simulink library "ssc_Probes_2016a_org"  (Simulink 10.0)
settings: Solver=ode45  StartTime=0.0  StopTime=10.0  RelTol=1e-3  EnableMultiTasking=on
libraries: fl_lib x64, nesl_utility x64, pe_lib x9
(part 3 of 3)

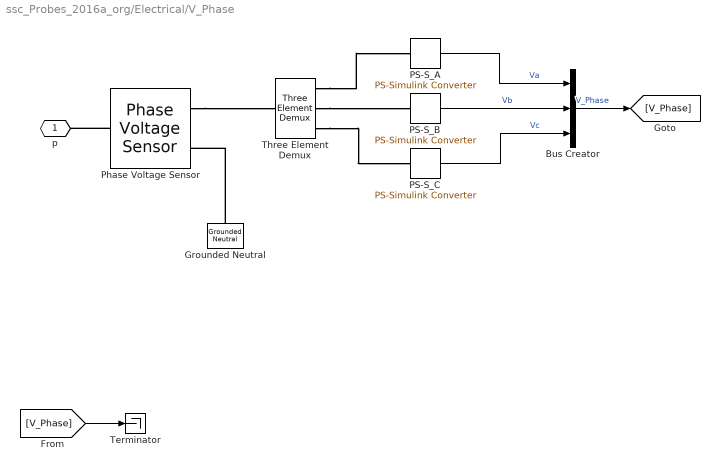
== system ssc_Probes_2016a_org/Electrical/V_Phase ==
  Bus Creator : BusCreator  Inputs=3
  Grounded Neutral : pe_lib/Connections/Grounded Neutral
      settings: SourceProductName=Simscape Electrical  SourceProductBaseCode=PS
  PS-S_A : nesl_utility/PS-Simulink Converter  PhysicalDomain=network_engine_domain  SubClassName=ps_output  LeftPortType=input  RightPortType=output  PseudoPeriodic=off  Frequencies=[]  Unit=V  AffineConversion=off
  PS-S_B : nesl_utility/PS-Simulink Converter  PhysicalDomain=network_engine_domain  SubClassName=ps_output  LeftPortType=input  RightPortType=output  PseudoPeriodic=off  Frequencies=[]  Unit=V  AffineConversion=off
  PS-S_C : nesl_utility/PS-Simulink Converter  PhysicalDomain=network_engine_domain  SubClassName=ps_output  LeftPortType=input  RightPortType=output  PseudoPeriodic=off  Frequencies=[]  Unit=V  AffineConversion=off
  Phase Voltage Sensor : pe_lib/Sensors/Phase Voltage Sensor
      settings: SourceProductName=Simscape Electrical  SourceProductBaseCode=PS
  Terminator : Terminator
  Three Element Demux : pe_lib/Sensors/Three Element Demux
      settings: SourceProductName=Simscape Electrical  SourceProductBaseCode=PS
  p : PMIOPort  Side=Left
  wires:
  [V_Phase] -> Terminator/1
  PS-S_A/1 -> Bus Creator/1  "Va"
  PS-S_B/1 -> Bus Creator/2  "Vb"
  PS-S_C/1 -> Bus Creator/3  "Vc"
  Bus Creator/1 -> [V_Phase]  "V_Phase"
  connections:
  Phase Voltage Sensor/LConn1 -- p/RConn1
  Three Element Demux/RConn3 -- PS-S_C/LConn1
  Three Element Demux/RConn1 -- PS-S_A/LConn1
  Three Element Demux/RConn2 -- PS-S_B/LConn1
  Phase Voltage Sensor/RConn1 -- Three Element Demux/LConn1
  Grounded Neutral/LConn1 -- Phase Voltage Sensor/RConn2

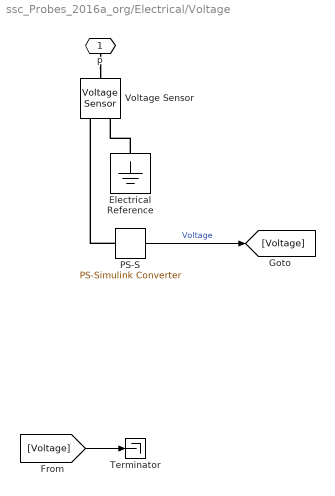
== system ssc_Probes_2016a_org/Electrical/Voltage ==
  Electrical Reference : fl_lib/Electrical/Electrical Elements/Electrical Reference
  PS-S : nesl_utility/PS-Simulink Converter  PhysicalDomain=network_engine_domain  SubClassName=ps_output  LeftPortType=input  RightPortType=output  PseudoPeriodic=off  Frequencies=[]  Unit=V  AffineConversion=off
  Terminator : Terminator
  Voltage Sensor : fl_lib/Electrical/Electrical Sensors/Voltage Sensor
  p : PMIOPort  Side=Left
  wires:
  PS-S/1 -> [Voltage]  "Voltage"
  [Voltage] -> Terminator/1
  connections:
  Electrical Reference/LConn1 -- Voltage Sensor/RConn2
  PS-S/LConn1 -- Voltage Sensor/RConn1
  p/RConn1 -- Voltage Sensor/LConn1

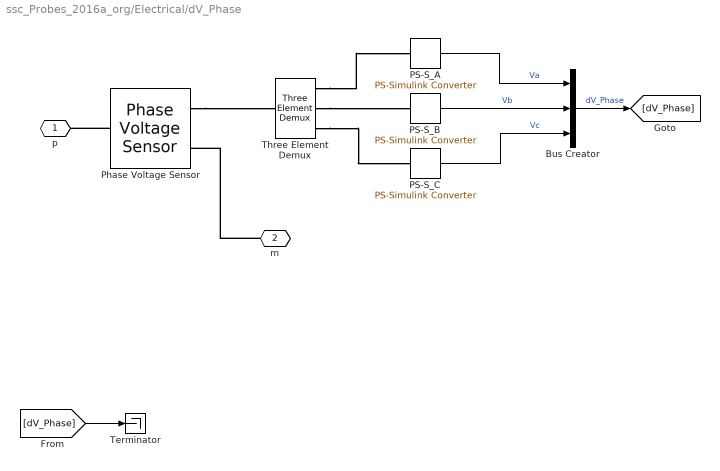
== system ssc_Probes_2016a_org/Electrical/dV_Phase ==
  Bus Creator : BusCreator  Inputs=3
  PS-S_A : nesl_utility/PS-Simulink Converter  PhysicalDomain=network_engine_domain  SubClassName=ps_output  LeftPortType=input  RightPortType=output  PseudoPeriodic=off  Frequencies=[]  Unit=V  AffineConversion=off
  PS-S_B : nesl_utility/PS-Simulink Converter  PhysicalDomain=network_engine_domain  SubClassName=ps_output  LeftPortType=input  RightPortType=output  PseudoPeriodic=off  Frequencies=[]  Unit=V  AffineConversion=off
  PS-S_C : nesl_utility/PS-Simulink Converter  PhysicalDomain=network_engine_domain  SubClassName=ps_output  LeftPortType=input  RightPortType=output  PseudoPeriodic=off  Frequencies=[]  Unit=V  AffineConversion=off
  Phase Voltage Sensor : pe_lib/Sensors/Phase Voltage Sensor
      settings: SourceProductName=Simscape Electrical  SourceProductBaseCode=PS
  Terminator : Terminator
  Three Element Demux : pe_lib/Sensors/Three Element Demux
      settings: SourceProductName=Simscape Electrical  SourceProductBaseCode=PS
  p : PMIOPort  Side=Left
  m : PMIOPort  Port=2  Side=Right
  wires:
  Bus Creator/1 -> [dV_Phase]  "dV_Phase"
  PS-S_C/1 -> Bus Creator/3  "Vc"
  PS-S_B/1 -> Bus Creator/2  "Vb"
  PS-S_A/1 -> Bus Creator/1  "Va"
  [dV_Phase] -> Terminator/1
  connections:
  m/RConn1 -- Phase Voltage Sensor/RConn2
  Phase Voltage Sensor/RConn1 -- Three Element Demux/LConn1
  Three Element Demux/RConn2 -- PS-S_B/LConn1
  Three Element Demux/RConn1 -- PS-S_A/LConn1
  Three Element Demux/RConn3 -- PS-S_C/LConn1
  Phase Voltage Sensor/LConn1 -- p/RConn1

== system ssc_Probes_2016a_org/Electrical/dVoltage ==
  PS-S : nesl_utility/PS-Simulink Converter  PhysicalDomain=network_engine_domain  SubClassName=ps_output  LeftPortType=input  RightPortType=output  PseudoPeriodic=off  Frequencies=[]  Unit=V  AffineConversion=off
  Terminator : Terminator
  Voltage Sensor : fl_lib/Electrical/Electrical Sensors/Voltage Sensor
  p : PMIOPort  Side=Left
  m : PMIOPort  Port=2  Side=Right
  wires:
  PS-S/1 -> [dVoltage]  "dVoltage"
  [dVoltage] -> Terminator/1
  connections:
  p/RConn1 -- Voltage Sensor/LConn1
  PS-S/LConn1 -- Voltage Sensor/RConn1
  m/RConn1 -- Voltage Sensor/RConn2

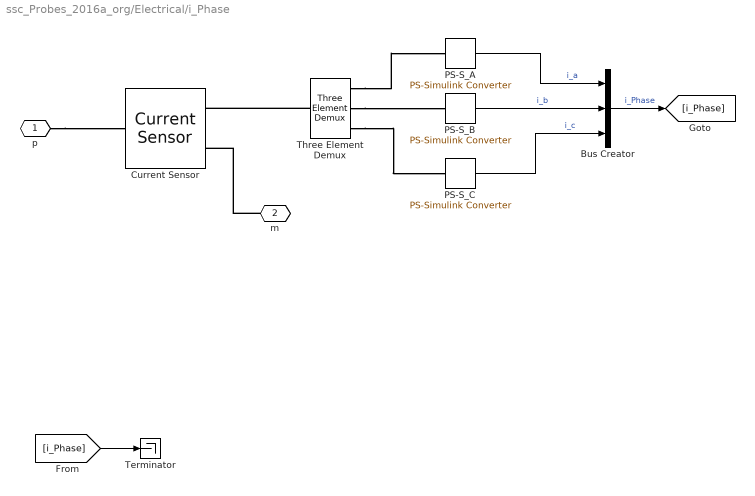
== system ssc_Probes_2016a_org/Electrical/i_Phase ==
  Bus Creator : BusCreator  Inputs=3
  Current Sensor : pe_lib/Sensors/Current Sensor
      settings: SourceProductName=Simscape Electrical  SourceProductBaseCode=PS
  PS-S_A : nesl_utility/PS-Simulink Converter  PhysicalDomain=network_engine_domain  SubClassName=ps_output  LeftPortType=input  RightPortType=output  PseudoPeriodic=off  Frequencies=[]  Unit=A  AffineConversion=off
  PS-S_B : nesl_utility/PS-Simulink Converter  PhysicalDomain=network_engine_domain  SubClassName=ps_output  LeftPortType=input  RightPortType=output  PseudoPeriodic=off  Frequencies=[]  Unit=A  AffineConversion=off
  PS-S_C : nesl_utility/PS-Simulink Converter  PhysicalDomain=network_engine_domain  SubClassName=ps_output  LeftPortType=input  RightPortType=output  PseudoPeriodic=off  Frequencies=[]  Unit=A  AffineConversion=off
  Terminator : Terminator
  Three Element Demux : pe_lib/Sensors/Three Element Demux
      settings: SourceProductName=Simscape Electrical  SourceProductBaseCode=PS
  p : PMIOPort  Side=Left
  m : PMIOPort  Port=2  Side=Right
  wires:
  [i_Phase] -> Terminator/1
  PS-S_A/1 -> Bus Creator/1  "i_a"
  PS-S_B/1 -> Bus Creator/2  "i_b"
  PS-S_C/1 -> Bus Creator/3  "i_c"
  Bus Creator/1 -> [i_Phase]  "i_Phase"
  connections:
  m/RConn1 -- Current Sensor/RConn2
  p/RConn1 -- Current Sensor/LConn1
  Three Element Demux/RConn3 -- PS-S_C/LConn1
  Three Element Demux/RConn2 -- PS-S_B/LConn1
  Three Element Demux/RConn1 -- PS-S_A/LConn1
  Three Element Demux/LConn1 -- Current Sensor/RConn1

== system ssc_Probes_2016a_org/Hydraulic/Flow ==
  Ideal Hydraulic Flow Rate Sensor : fl_lib/Hydraulic/Hydraulic Sensors/Hydraulic Flow Rate Sensor
      settings: SourceProductName=Simscape
  PS-S : nesl_utility/PS-Simulink Converter  PhysicalDomain=network_engine_domain  SubClassName=ps_output  LeftPortType=input  RightPortType=output  PseudoPeriodic=off  Frequencies=[]  Unit=m^3/s  AffineConversion=off
  Terminator : Terminator
  A : PMIOPort  Side=Left
  B : PMIOPort  Port=2  Side=Right
  wires:
  PS-S/1 -> [Flow]  "Flow"
  [Flow] -> Terminator/1
  connections:
  B/RConn1 -- Ideal Hydraulic Flow Rate Sensor/RConn2
  Ideal Hydraulic Flow Rate Sensor/RConn1 -- PS-S/LConn1
  A/RConn1 -- Ideal Hydraulic Flow Rate Sensor/LConn1

== system ssc_Probes_2016a_org/Hydraulic/Pressure ==
  Hydraulic Reference : fl_lib/Hydraulic/Hydraulic Elements/Hydraulic Reference
      settings: SourceProductName=Simscape
  Ideal Hydraulic Pressure Sensor : fl_lib/Hydraulic/Hydraulic Sensors/Hydraulic Pressure Sensor
      settings: SourceProductName=Simscape
  PS-S : nesl_utility/PS-Simulink Converter  PhysicalDomain=network_engine_domain  SubClassName=ps_output  LeftPortType=input  RightPortType=output  PseudoPeriodic=off  Frequencies=[]  Unit=Pa  AffineConversion=off
  Terminator : Terminator
  A : PMIOPort  Side=Left
  wires:
  PS-S/1 -> [Pressure]  "Pressure"
  [Pressure] -> Terminator/1
  connections:
  PS-S/LConn1 -- Ideal Hydraulic Pressure Sensor/RConn2
  Hydraulic Reference/LConn1 -- Ideal Hydraulic Pressure Sensor/RConn1
  A/RConn1 -- Ideal Hydraulic Pressure Sensor/LConn1

== system ssc_Probes_2016a_org/Hydraulic/dPressure ==
  Ideal Hydraulic Pressure Sensor : fl_lib/Hydraulic/Hydraulic Sensors/Hydraulic Pressure Sensor
      settings: SourceProductName=Simscape
  PS-S : nesl_utility/PS-Simulink Converter  PhysicalDomain=network_engine_domain  SubClassName=ps_output  LeftPortType=input  RightPortType=output  PseudoPeriodic=off  Frequencies=[]  Unit=Pa  AffineConversion=off
  Terminator : Terminator
  A : PMIOPort  Side=Left
  B : PMIOPort  Port=2  Side=Right
  wires:
  PS-S/1 -> [dPressure]  "dPressure"
  [dPressure] -> Terminator/1
  connections:
  A/RConn1 -- Ideal Hydraulic Pressure Sensor/LConn1
  B/RConn1 -- Ideal Hydraulic Pressure Sensor/RConn1
  PS-S/LConn1 -- Ideal Hydraulic Pressure Sensor/RConn2

== system ssc_Probes_2016a_org/Magnetic/Flux ==
  Flux Sensor : fl_lib/Magnetic/Magnetic Sensors/Flux Sensor
      settings: SourceProductName=Simscape  SourceProductBaseCode=SS
  PS-S : nesl_utility/PS-Simulink Converter  PhysicalDomain=network_engine_domain  SubClassName=ps_output  LeftPortType=input  RightPortType=output  PseudoPeriodic=off  Frequencies=[]  Unit=Wb  AffineConversion=off
  Terminator : Terminator
  N : PMIOPort  Side=Left
  S : PMIOPort  Port=2  Side=Right
  wires:
  PS-S/1 -> [Flux]  "Flux"
  [Flux] -> Terminator/1
  connections:
  N/RConn1 -- Flux Sensor/LConn1
  Flux Sensor/RConn1 -- PS-S/LConn1
  S/RConn1 -- Flux Sensor/RConn2

== system ssc_Probes_2016a_org/Magnetic/MMF ==
  MMF Sensor : fl_lib/Magnetic/Magnetic Sensors/MMF Sensor
      settings: SourceProductName=Simscape  SourceProductBaseCode=SS
  Magnetic Reference : fl_lib/Magnetic/Magnetic Elements/Magnetic Reference
      settings: SourceProductName=Simscape  SourceProductBaseCode=SS
  PS-S : nesl_utility/PS-Simulink Converter  PhysicalDomain=network_engine_domain  SubClassName=ps_output  LeftPortType=input  RightPortType=output  PseudoPeriodic=off  Frequencies=[]  Unit=A  AffineConversion=off
  Terminator : Terminator
  N : PMIOPort  Side=Left
  wires:
  PS-S/1 -> [MMF]  "MMF"
  [MMF] -> Terminator/1
  connections:
  Magnetic Reference/LConn1 -- MMF Sensor/RConn2
  MMF Sensor/RConn1 -- PS-S/LConn1
  N/RConn1 -- MMF Sensor/LConn1

== system ssc_Probes_2016a_org/Magnetic/dMMF ==
  MMF Sensor : fl_lib/Magnetic/Magnetic Sensors/MMF Sensor
      settings: SourceProductName=Simscape  SourceProductBaseCode=SS
  PS-S : nesl_utility/PS-Simulink Converter  PhysicalDomain=network_engine_domain  SubClassName=ps_output  LeftPortType=input  RightPortType=output  PseudoPeriodic=off  Frequencies=[]  Unit=A  AffineConversion=off
  Terminator : Terminator
  N : PMIOPort  Side=Left
  S : PMIOPort  Port=2  Side=Right
  wires:
  PS-S/1 -> [dMMF]  "dMMF"
  [dMMF] -> Terminator/1
  connections:
  N/RConn1 -- MMF Sensor/LConn1
  MMF Sensor/RConn1 -- PS-S/LConn1
  S/RConn1 -- MMF Sensor/RConn2

== system ssc_Probes_2016a_org/Mechanical/AngVel ==
  Ideal Rotational Motion Sensor : fl_lib/Mechanical/Mechanical Sensors/Ideal Rotational Motion Sensor  offset=0 rad
  Mechanical Rotational Reference : fl_lib/Mechanical/Rotational Elements/Mechanical Rotational Reference
  PS-S : nesl_utility/PS-Simulink Converter  PhysicalDomain=network_engine_domain  SubClassName=ps_output  LeftPortType=input  RightPortType=output  PseudoPeriodic=off  Frequencies=[]  Unit=rad/s  AffineConversion=off
  Terminator : Terminator
  R : PMIOPort  Side=Left
  wires:
  PS-S/1 -> [AngVel]  "AngVel"
  [AngVel] -> Terminator/1
  connections:
  Ideal Rotational Motion Sensor/RConn2 -- PS-S/LConn1
  Mechanical Rotational Reference/LConn1 -- Ideal Rotational Motion Sensor/RConn1
  R/RConn1 -- Ideal Rotational Motion Sensor/LConn1

== system ssc_Probes_2016a_org/Mechanical/Angle ==
  Ideal Rotational Motion Sensor : fl_lib/Mechanical/Mechanical Sensors/Ideal Rotational Motion Sensor  offset=0 rad
  Mechanical Rotational Reference : fl_lib/Mechanical/Rotational Elements/Mechanical Rotational Reference
  PS-S : nesl_utility/PS-Simulink Converter  PhysicalDomain=network_engine_domain  SubClassName=ps_output  LeftPortType=input  RightPortType=output  PseudoPeriodic=off  Frequencies=[]  Unit=rad  AffineConversion=off
  Terminator : Terminator
  R : PMIOPort  Side=Left
  wires:
  PS-S/1 -> [Angle]  "Angle"
  [Angle] -> Terminator/1
  connections:
  R/RConn1 -- Ideal Rotational Motion Sensor/LConn1
  Mechanical Rotational Reference/LConn1 -- Ideal Rotational Motion Sensor/RConn1
  PS-S/LConn1 -- Ideal Rotational Motion Sensor/RConn3

== system ssc_Probes_2016a_org/Mechanical/Force ==
  Ideal Force Sensor : fl_lib/Mechanical/Mechanical Sensors/Ideal Force Sensor
  PS-S : nesl_utility/PS-Simulink Converter  PhysicalDomain=network_engine_domain  SubClassName=ps_output  LeftPortType=input  RightPortType=output  PseudoPeriodic=off  Frequencies=[]  Unit=N  AffineConversion=off
  Terminator : Terminator
  R : PMIOPort  Side=Left
  C : PMIOPort  Port=2  Side=Right
  wires:
  PS-S/1 -> [Force]  "Force"
  [Force] -> Terminator/1
  connections:
  C/RConn1 -- Ideal Force Sensor/RConn1
  Ideal Force Sensor/RConn2 -- PS-S/LConn1
  R/RConn1 -- Ideal Force Sensor/LConn1

== system ssc_Probes_2016a_org/Mechanical/Position ==
  Ideal Translational Motion Sensor : fl_lib/Mechanical/Mechanical Sensors/Ideal Translational Motion Sensor  offset=0 m
  Mechanical Translational Reference : fl_lib/Mechanical/Translational Elements/Mechanical Translational Reference
  PS-S : nesl_utility/PS-Simulink Converter  PhysicalDomain=network_engine_domain  SubClassName=ps_output  LeftPortType=input  RightPortType=output  PseudoPeriodic=off  Frequencies=[]  Unit=m  AffineConversion=off
  Terminator : Terminator
  R : PMIOPort  Side=Left
  wires:
  PS-S/1 -> [Position]  "Position"
  [Position] -> Terminator/1
  connections:
  PS-S/LConn1 -- Ideal Translational Motion Sensor/RConn3
  Mechanical Translational Reference/LConn1 -- Ideal Translational Motion Sensor/RConn1
  R/RConn1 -- Ideal Translational Motion Sensor/LConn1

== system ssc_Probes_2016a_org/Mechanical/Torque ==
  Ideal Torque Sensor : fl_lib/Mechanical/Mechanical Sensors/Ideal Torque Sensor
  PS-S : nesl_utility/PS-Simulink Converter  PhysicalDomain=network_engine_domain  SubClassName=ps_output  LeftPortType=input  RightPortType=output  PseudoPeriodic=off  Frequencies=[]  Unit=N*m  AffineConversion=off
  Terminator : Terminator
  R : PMIOPort  Side=Left
  C : PMIOPort  Port=2  Side=Right
  wires:
  PS-S/1 -> [Torque]  "Torque"
  [Torque] -> Terminator/1
  connections:
  R/RConn1 -- Ideal Torque Sensor/LConn1
  Ideal Torque Sensor/RConn2 -- PS-S/LConn1
  C/RConn1 -- Ideal Torque Sensor/RConn1

== system ssc_Probes_2016a_org/Mechanical/Velocity ==
  Ideal Translational Motion Sensor : fl_lib/Mechanical/Mechanical Sensors/Ideal Translational Motion Sensor  offset=0 m
  Mechanical Translational Reference : fl_lib/Mechanical/Translational Elements/Mechanical Translational Reference
  PS-S : nesl_utility/PS-Simulink Converter  PhysicalDomain=network_engine_domain  SubClassName=ps_output  LeftPortType=input  RightPortType=output  PseudoPeriodic=off  Frequencies=[]  Unit=m/s  AffineConversion=off
  Terminator : Terminator
  R : PMIOPort  Side=Left
  wires:
  PS-S/1 -> [Velocity]  "Velocity"
  [Velocity] -> Terminator/1
  connections:
  Ideal Translational Motion Sensor/RConn2 -- PS-S/LConn1
  R/RConn1 -- Ideal Translational Motion Sensor/LConn1
  Mechanical Translational Reference/LConn1 -- Ideal Translational Motion Sensor/RConn1

== system ssc_Probes_2016a_org/Mechanical/dAngVel ==
  Ideal Rotational Motion Sensor : fl_lib/Mechanical/Mechanical Sensors/Ideal Rotational Motion Sensor  offset=0 rad
  PS-S : nesl_utility/PS-Simulink Converter  PhysicalDomain=network_engine_domain  SubClassName=ps_output  LeftPortType=input  RightPortType=output  PseudoPeriodic=off  Frequencies=[]  Unit=rad/s  AffineConversion=off
  Terminator : Terminator
  R : PMIOPort  Side=Left
  C : PMIOPort  Port=2  Side=Right
  wires:
  PS-S/1 -> [dAngVel]  "dAngVel"
  [dAngVel] -> Terminator/1
  connections:
  R/RConn1 -- Ideal Rotational Motion Sensor/LConn1
  C/RConn1 -- Ideal Rotational Motion Sensor/RConn1
  Ideal Rotational Motion Sensor/RConn2 -- PS-S/LConn1

== system ssc_Probes_2016a_org/Mechanical/dAngle ==
  Ideal Rotational Motion Sensor : fl_lib/Mechanical/Mechanical Sensors/Ideal Rotational Motion Sensor  offset=0 rad
  PS-S : nesl_utility/PS-Simulink Converter  PhysicalDomain=network_engine_domain  SubClassName=ps_output  LeftPortType=input  RightPortType=output  PseudoPeriodic=off  Frequencies=[]  Unit=rad  AffineConversion=off
  Terminator : Terminator
  R : PMIOPort  Side=Left
  C : PMIOPort  Port=2  Side=Right
  wires:
  PS-S/1 -> [dAngle]  "dAngle"
  [dAngle] -> Terminator/1
  connections:
  PS-S/LConn1 -- Ideal Rotational Motion Sensor/RConn3
  C/RConn1 -- Ideal Rotational Motion Sensor/RConn1
  R/RConn1 -- Ideal Rotational Motion Sensor/LConn1

== system ssc_Probes_2016a_org/Mechanical/dPosition ==
  Ideal Translational Motion Sensor : fl_lib/Mechanical/Mechanical Sensors/Ideal Translational Motion Sensor  offset=0 m
  PS-S : nesl_utility/PS-Simulink Converter  PhysicalDomain=network_engine_domain  SubClassName=ps_output  LeftPortType=input  RightPortType=output  PseudoPeriodic=off  Frequencies=[]  Unit=m  AffineConversion=off
  Terminator : Terminator
  R : PMIOPort  Side=Left
  C : PMIOPort  Port=2  Side=Right
  wires:
  PS-S/1 -> [dPosition]  "dPosition"
  [dPosition] -> Terminator/1
  connections:
  R/RConn1 -- Ideal Translational Motion Sensor/LConn1
  C/RConn1 -- Ideal Translational Motion Sensor/RConn1
  PS-S/LConn1 -- Ideal Translational Motion Sensor/RConn3

== system ssc_Probes_2016a_org/Mechanical/dVelocity ==
  Ideal Translational Motion Sensor : fl_lib/Mechanical/Mechanical Sensors/Ideal Translational Motion Sensor  offset=0 m
  PS-S : nesl_utility/PS-Simulink Converter  PhysicalDomain=network_engine_domain  SubClassName=ps_output  LeftPortType=input  RightPortType=output  PseudoPeriodic=off  Frequencies=[]  Unit=m/s  AffineConversion=off
  Terminator : Terminator
  R : PMIOPort  Side=Left
  C : PMIOPort  Port=2  Side=Right
  wires:
  PS-S/1 -> [dVelocity]  "dVelocity"
  [dVelocity] -> Terminator/1
  connections:
  C/RConn1 -- Ideal Translational Motion Sensor/RConn1
  R/RConn1 -- Ideal Translational Motion Sensor/LConn1
  PS-S/LConn1 -- Ideal Translational Motion Sensor/RConn2

== system ssc_Probes_2016a_org/Pneumatic/AbsPressure ==
  PS-S : nesl_utility/PS-Simulink Converter  PhysicalDomain=network_engine_domain  SubClassName=ps_output  LeftPortType=input  RightPortType=output  PseudoPeriodic=off  Frequencies=[]  Unit=Pa  AffineConversion=off
  Pneumatic Absolute Reference : fl_lib/Pneumatic/Pneumatic Elements/Pneumatic Absolute Reference
      settings: SourceProductName=Simscape  SourceProductBaseCode=SS
  Pneumatic Pressure & Temperature Sensor : fl_lib/Pneumatic/Pneumatic Sensors/Pneumatic Pressure & Temperature Sensor
      settings: SourceProductName=Simscape  SourceProductBaseCode=SS
  Terminator : Terminator
  A : PMIOPort  Side=Left
  wires:
  PS-S/1 -> [AbsPressure]  "AbsPressure"
  [AbsPressure] -> Terminator/1
  connections:
  A/RConn1 -- Pneumatic Pressure & Temperature Sensor/LConn1
  Pneumatic Absolute Reference/LConn1 -- Pneumatic Pressure & Temperature Sensor/RConn1
  PS-S/LConn1 -- Pneumatic Pressure & Temperature Sensor/RConn2

== system ssc_Probes_2016a_org/Pneumatic/AbsTemperature ==
  PS-S : nesl_utility/PS-Simulink Converter  PhysicalDomain=network_engine_domain  SubClassName=ps_output  LeftPortType=input  RightPortType=output  PseudoPeriodic=off  Frequencies=[]  Unit=K  AffineConversion=off
  Pneumatic Absolute Reference : fl_lib/Pneumatic/Pneumatic Elements/Pneumatic Absolute Reference
      settings: SourceProductName=Simscape  SourceProductBaseCode=SS
  Pneumatic Pressure & Temperature Sensor : fl_lib/Pneumatic/Pneumatic Sensors/Pneumatic Pressure & Temperature Sensor
      settings: SourceProductName=Simscape  SourceProductBaseCode=SS
  Terminator : Terminator
  A : PMIOPort  Side=Left
  wires:
  PS-S/1 -> [AbsTemperature]  "AbsTemperature"
  [AbsTemperature] -> Terminator/1
  connections:
  PS-S/LConn1 -- Pneumatic Pressure & Temperature Sensor/RConn3
  Pneumatic Absolute Reference/LConn1 -- Pneumatic Pressure & Temperature Sensor/RConn1
  A/RConn1 -- Pneumatic Pressure & Temperature Sensor/LConn1

== system ssc_Probes_2016a_org/Pneumatic/AtmTemperature ==
  PS-S : nesl_utility/PS-Simulink Converter  PhysicalDomain=network_engine_domain  SubClassName=ps_output  LeftPortType=input  RightPortType=output  PseudoPeriodic=off  Frequencies=[]  Unit=K  AffineConversion=off
  Pneumatic Atmospheric Reference : fl_lib/Pneumatic/Pneumatic Elements/Pneumatic Atmospheric Reference
      settings: SourceProductName=Simscape  SourceProductBaseCode=SS
  Pneumatic Pressure & Temperature Sensor : fl_lib/Pneumatic/Pneumatic Sensors/Pneumatic Pressure & Temperature Sensor
      settings: SourceProductName=Simscape  SourceProductBaseCode=SS
  Terminator : Terminator
  A : PMIOPort  Side=Left
  wires:
  PS-S/1 -> [AtmTemperature]  "AtmTemperature"
  [AtmTemperature] -> Terminator/1
  connections:
  A/RConn1 -- Pneumatic Pressure & Temperature Sensor/LConn1
  Pneumatic Atmospheric Reference/LConn1 -- Pneumatic Pressure & Temperature Sensor/RConn1
  PS-S/LConn1 -- Pneumatic Pressure & Temperature Sensor/RConn3

== system ssc_Probes_2016a_org/Pneumatic/GasHeatFlow ==
  PS-S : nesl_utility/PS-Simulink Converter  PhysicalDomain=network_engine_domain  SubClassName=ps_output  LeftPortType=input  RightPortType=output  PseudoPeriodic=off  Frequencies=[]  Unit=J/s  AffineConversion=off
  Pneumatic Mass & Heat Flow Sensor : fl_lib/Pneumatic/Pneumatic Sensors/Pneumatic Mass & Heat Flow Sensor
      settings: SourceProductName=Simscape  SourceProductBaseCode=SS
  Terminator : Terminator
  A : PMIOPort  Side=Left
  B : PMIOPort  Port=2  Side=Right
  wires:
  PS-S/1 -> [GasHeatFlow]  "GasHeatFlow"
  [GasHeatFlow] -> Terminator/1
  connections:
  PS-S/LConn1 -- Pneumatic Mass & Heat Flow Sensor/RConn3
  B/RConn1 -- Pneumatic Mass & Heat Flow Sensor/RConn1
  A/RConn1 -- Pneumatic Mass & Heat Flow Sensor/LConn1

== system ssc_Probes_2016a_org/Pneumatic/GaugePressure ==
  PS-S : nesl_utility/PS-Simulink Converter  PhysicalDomain=network_engine_domain  SubClassName=ps_output  LeftPortType=input  RightPortType=output  PseudoPeriodic=off  Frequencies=[]  Unit=Pa  AffineConversion=off
  Pneumatic Atmospheric Reference : fl_lib/Pneumatic/Pneumatic Elements/Pneumatic Atmospheric Reference
      settings: SourceProductName=Simscape  SourceProductBaseCode=SS
  Pneumatic Pressure & Temperature Sensor : fl_lib/Pneumatic/Pneumatic Sensors/Pneumatic Pressure & Temperature Sensor
      settings: SourceProductName=Simscape  SourceProductBaseCode=SS
  Terminator : Terminator
  A : PMIOPort  Side=Left
  wires:
  PS-S/1 -> [GaugePressure]  "GaugePressure"
  [GaugePressure] -> Terminator/1
  connections:
  PS-S/LConn1 -- Pneumatic Pressure & Temperature Sensor/RConn2
  Pneumatic Atmospheric Reference/LConn1 -- Pneumatic Pressure & Temperature Sensor/RConn1
  A/RConn1 -- Pneumatic Pressure & Temperature Sensor/LConn1

== system ssc_Probes_2016a_org/Pneumatic/MassFlow ==
  PS-S : nesl_utility/PS-Simulink Converter  PhysicalDomain=network_engine_domain  SubClassName=ps_output  LeftPortType=input  RightPortType=output  PseudoPeriodic=off  Frequencies=[]  Unit=kg/s  AffineConversion=off
  Pneumatic Mass & Heat Flow Sensor : fl_lib/Pneumatic/Pneumatic Sensors/Pneumatic Mass & Heat Flow Sensor
      settings: SourceProductName=Simscape  SourceProductBaseCode=SS
  Terminator : Terminator
  A : PMIOPort  Side=Left
  B : PMIOPort  Port=2  Side=Right
  wires:
  PS-S/1 -> [MassFlow]  "MassFlow"
  [MassFlow] -> Terminator/1
  connections:
  A/RConn1 -- Pneumatic Mass & Heat Flow Sensor/LConn1
  Pneumatic Mass & Heat Flow Sensor/RConn2 -- PS-S/LConn1
  B/RConn1 -- Pneumatic Mass & Heat Flow Sensor/RConn1

== system ssc_Probes_2016a_org/Pneumatic/dGasPressure ==
  PS-S : nesl_utility/PS-Simulink Converter  PhysicalDomain=network_engine_domain  SubClassName=ps_output  LeftPortType=input  RightPortType=output  PseudoPeriodic=off  Frequencies=[]  Unit=Pa  AffineConversion=off
  Pneumatic Pressure & Temperature Sensor : fl_lib/Pneumatic/Pneumatic Sensors/Pneumatic Pressure & Temperature Sensor
      settings: SourceProductName=Simscape  SourceProductBaseCode=SS
  Terminator : Terminator
  A : PMIOPort  Side=Left
  B : PMIOPort  Port=2  Side=Right
  wires:
  PS-S/1 -> [dGasPressure]  "dGasPressure"
  [dGasPressure] -> Terminator/1
  connections:
  A/RConn1 -- Pneumatic Pressure & Temperature Sensor/LConn1
  B/RConn1 -- Pneumatic Pressure & Temperature Sensor/RConn1
  Pneumatic Pressure & Temperature Sensor/RConn2 -- PS-S/LConn1

== system ssc_Probes_2016a_org/Pneumatic/dGasTemperature ==
  PS-S : nesl_utility/PS-Simulink Converter  PhysicalDomain=network_engine_domain  SubClassName=ps_output  LeftPortType=input  RightPortType=output  PseudoPeriodic=off  Frequencies=[]  Unit=K  AffineConversion=off
  Pneumatic Pressure & Temperature Sensor : fl_lib/Pneumatic/Pneumatic Sensors/Pneumatic Pressure & Temperature Sensor
      settings: SourceProductName=Simscape  SourceProductBaseCode=SS
  Terminator : Terminator
  A : PMIOPort  Side=Left
  B : PMIOPort  Port=2  Side=Right
  wires:
  PS-S/1 -> [dGasTemperature]  "dGasTemperature"
  [dGasTemperature] -> Terminator/1
  connections:
  PS-S/LConn1 -- Pneumatic Pressure & Temperature Sensor/RConn3
  B/RConn1 -- Pneumatic Pressure & Temperature Sensor/RConn1
  A/RConn1 -- Pneumatic Pressure & Temperature Sensor/LConn1

== system ssc_Probes_2016a_org/Thermal/HeatFlow ==
  Ideal Heat Flow Sensor : fl_lib/Thermal/Thermal Sensors/Ideal Heat Flow Sensor
      settings: SourceProductName=Simscape  SourceProductBaseCode=SS
  PS-S : nesl_utility/PS-Simulink Converter  PhysicalDomain=network_engine_domain  SubClassName=ps_output  LeftPortType=input  RightPortType=output  PseudoPeriodic=off  Frequencies=[]  Unit=J/s  AffineConversion=off
  Terminator : Terminator
  A : PMIOPort  Side=Left
  B : PMIOPort  Port=2  Side=Right
  wires:
  PS-S/1 -> [HeatFlow]  "HeatFlow"
  [HeatFlow] -> Terminator/1
  connections:
  A/RConn1 -- Ideal Heat Flow Sensor/LConn1
  Ideal Heat Flow Sensor/RConn1 -- PS-S/LConn1
  B/RConn1 -- Ideal Heat Flow Sensor/RConn2

== system ssc_Probes_2016a_org/Thermal/Temperature ==
  Ideal Temperature Sensor : fl_lib/Thermal/Thermal Sensors/Ideal Temperature Sensor
      settings: SourceProductName=Simscape  SourceProductBaseCode=SS
  PS-S : nesl_utility/PS-Simulink Converter  PhysicalDomain=network_engine_domain  SubClassName=ps_output  LeftPortType=input  RightPortType=output  PseudoPeriodic=off  Frequencies=[]  Unit=K  AffineConversion=off
  Terminator : Terminator
  Thermal Reference : fl_lib/Thermal/Thermal Elements/Thermal Reference
  A : PMIOPort  Side=Left
  wires:
  PS-S/1 -> [Temperature]  "Temperature"
  [Temperature] -> Terminator/1
  connections:
  A/RConn1 -- Ideal Temperature Sensor/LConn1
  Thermal Reference/LConn1 -- Ideal Temperature Sensor/RConn1
  PS-S/LConn1 -- Ideal Temperature Sensor/RConn2

== system ssc_Probes_2016a_org/Thermal/dTemperature ==
  Ideal Temperature Sensor : fl_lib/Thermal/Thermal Sensors/Ideal Temperature Sensor
      settings: SourceProductName=Simscape  SourceProductBaseCode=SS
  PS-S : nesl_utility/PS-Simulink Converter  PhysicalDomain=network_engine_domain  SubClassName=ps_output  LeftPortType=input  RightPortType=output  PseudoPeriodic=off  Frequencies=[]  Unit=K  AffineConversion=off
  Terminator : Terminator
  A : PMIOPort  Side=Left
  B : PMIOPort  Port=2  Side=Right
  wires:
  PS-S/1 -> [dTemperature]  "dTemperature"
  [dTemperature] -> Terminator/1
  connections:
  PS-S/LConn1 -- Ideal Temperature Sensor/RConn2
  B/RConn1 -- Ideal Temperature Sensor/RConn1
  A/RConn1 -- Ideal Temperature Sensor/LConn1

== system ssc_Probes_2016a_org/ThermalLiquid/AbsPressure_TL ==
  Absolute Reference (TL) : fl_lib/Thermal Liquid/Elements/Absolute Reference (TL)
      settings: SourceProductName=Simscape  SourceProductBaseCode=SS
  PS-S : nesl_utility/PS-Simulink Converter  PhysicalDomain=network_engine_domain  SubClassName=ps_output  LeftPortType=input  RightPortType=output  PseudoPeriodic=off  Frequencies=[]  Unit=Pa  AffineConversion=off
  Pressure & Temperature Sensor (TL) : fl_lib/Thermal Liquid/Sensors/Pressure & Temperature Sensor (TL)
      settings: SourceProductName=Simscape  SourceProductBaseCode=SS
  Terminator : Terminator
  A : PMIOPort  Side=Left
  wires:
  PS-S/1 -> [AbsPressure_TL]  "AbsPressure_TL"
  [AbsPressure_TL] -> Terminator/1
  connections:
  Absolute Reference (TL)/LConn1 -- Pressure & Temperature Sensor (TL)/RConn1
  Pressure & Temperature Sensor (TL)/LConn1 -- A/RConn1
  PS-S/LConn1 -- Pressure & Temperature Sensor (TL)/RConn2

== system ssc_Probes_2016a_org/ThermalLiquid/AbsTemperature_TL ==
  Absolute Reference (TL) : fl_lib/Thermal Liquid/Elements/Absolute Reference (TL)
      settings: SourceProductName=Simscape  SourceProductBaseCode=SS
  PS-S : nesl_utility/PS-Simulink Converter  PhysicalDomain=network_engine_domain  SubClassName=ps_output  LeftPortType=input  RightPortType=output  PseudoPeriodic=off  Frequencies=[]  Unit=K  AffineConversion=off
  Pressure & Temperature Sensor (TL) : fl_lib/Thermal Liquid/Sensors/Pressure & Temperature Sensor (TL)
      settings: SourceProductName=Simscape  SourceProductBaseCode=SS
  Terminator : Terminator
  A : PMIOPort  Side=Left
  wires:
  [AbsTemperature_TL] -> Terminator/1
  PS-S/1 -> [AbsTemperature_TL]  "AbsTemperature_TL"
  connections:
  PS-S/LConn1 -- Pressure & Temperature Sensor (TL)/RConn3
  Pressure & Temperature Sensor (TL)/LConn1 -- A/RConn1
  Absolute Reference (TL)/LConn1 -- Pressure & Temperature Sensor (TL)/RConn1

== system ssc_Probes_2016a_org/ThermalLiquid/MassFlow_TL ==
  Mass Flow Rate & Thermal Flux Sensor (TL) : fl_lib/Thermal Liquid/Sensors/Mass & Energy Flow Rate Sensor (TL)
      settings: SourceProductName=Simscape  SourceProductBaseCode=SS
  PS-S : nesl_utility/PS-Simulink Converter  PhysicalDomain=network_engine_domain  SubClassName=ps_output  LeftPortType=input  RightPortType=output  PseudoPeriodic=off  Frequencies=[]  Unit=kg/s  AffineConversion=off
  Terminator : Terminator
  A : PMIOPort  Side=Left
  B : PMIOPort  Port=2  Side=Right
  wires:
  [MassFlow_TL] -> Terminator/1
  PS-S/1 -> [MassFlow_TL]  "MassFlow_TL"
  connections:
  Mass Flow Rate & Thermal Flux Sensor (TL)/RConn1 -- B/RConn1
  PS-S/LConn1 -- Mass Flow Rate & Thermal Flux Sensor (TL)/RConn2
  Mass Flow Rate & Thermal Flux Sensor (TL)/LConn1 -- A/RConn1

== system ssc_Probes_2016a_org/ThermalLiquid/ThermalFlux_TL ==
  Mass Flow Rate & Thermal Flux Sensor (TL) : fl_lib/Thermal Liquid/Sensors/Mass & Energy Flow Rate Sensor (TL)
      settings: SourceProductName=Simscape  SourceProductBaseCode=SS
  PS-S : nesl_utility/PS-Simulink Converter  PhysicalDomain=network_engine_domain  SubClassName=ps_output  LeftPortType=input  RightPortType=output  PseudoPeriodic=off  Frequencies=[]  Unit=J/s  AffineConversion=off
  Terminator : Terminator
  A : PMIOPort  Side=Left
  B : PMIOPort  Port=2  Side=Right
  wires:
  PS-S/1 -> [ThermalFlux_TL]  "ThermalFlux_TL"
  [ThermalFlux_TL] -> Terminator/1
  connections:
  Mass Flow Rate & Thermal Flux Sensor (TL)/LConn1 -- A/RConn1
  Mass Flow Rate & Thermal Flux Sensor (TL)/RConn1 -- B/RConn1
  Mass Flow Rate & Thermal Flux Sensor (TL)/RConn3 -- PS-S/LConn1

== system ssc_Probes_2016a_org/ThermalLiquid/dPressure_TL ==
  PS-S : nesl_utility/PS-Simulink Converter  PhysicalDomain=network_engine_domain  SubClassName=ps_output  LeftPortType=input  RightPortType=output  PseudoPeriodic=off  Frequencies=[]  Unit=Pa  AffineConversion=off
  Pressure & Temperature Sensor (TL) : fl_lib/Thermal Liquid/Sensors/Pressure & Temperature Sensor (TL)
      settings: SourceProductName=Simscape  SourceProductBaseCode=SS
  Terminator : Terminator
  A : PMIOPort  Side=Left
  B : PMIOPort  Port=2  Side=Right
  wires:
  PS-S/1 -> [dPressure_TL]  "dPressure_TL"
  [dPressure_TL] -> Terminator/1
  connections:
  B/RConn1 -- Pressure & Temperature Sensor (TL)/RConn1
  Pressure & Temperature Sensor (TL)/LConn1 -- A/RConn1
  Pressure & Temperature Sensor (TL)/RConn2 -- PS-S/LConn1

== system ssc_Probes_2016a_org/ThermalLiquid/dTemperature_TL ==
  PS-S : nesl_utility/PS-Simulink Converter  PhysicalDomain=network_engine_domain  SubClassName=ps_output  LeftPortType=input  RightPortType=output  PseudoPeriodic=off  Frequencies=[]  Unit=K  AffineConversion=off
  Pressure & Temperature Sensor (TL) : fl_lib/Thermal Liquid/Sensors/Pressure & Temperature Sensor (TL)
      settings: SourceProductName=Simscape  SourceProductBaseCode=SS
  Terminator : Terminator
  A : PMIOPort  Side=Left
  B : PMIOPort  Port=2  Side=Right
  wires:
  [dTemperature_TL] -> Terminator/1
  PS-S/1 -> [dTemperature_TL]  "dTemperature_TL"
  connections:
  Pressure & Temperature Sensor (TL)/LConn1 -- A/RConn1
  B/RConn1 -- Pressure & Temperature Sensor (TL)/RConn1
  PS-S/LConn1 -- Pressure & Temperature Sensor (TL)/RConn3

== system ssc_Probes_2016a_org/TwoPhaseFluid/AbsPressure_2P ==
  Absolute Reference (2P) : fl_lib/Two-Phase Fluid/Elements/Absolute Reference (2P)
      settings: SourceProductName=Simscape  SourceProductBaseCode=SS
  PS-S : nesl_utility/PS-Simulink Converter  PhysicalDomain=network_engine_domain  SubClassName=ps_output  LeftPortType=input  RightPortType=output  PseudoPeriodic=off  Frequencies=[]  Unit=Pa  AffineConversion=off
  Pressure & Internal Energy Sensor (2P) : fl_lib/Two-Phase Fluid/Sensors/Pressure & Internal Energy Sensor (2P)
      settings: SourceProductName=Simscape  SourceProductBaseCode=SS
  Terminator : Terminator
  A : PMIOPort  Side=Left
  wires:
  PS-S/1 -> [AbsPressure_2P]  "AbsPressure_2P"
  [AbsPressure_2P] -> Terminator/1
  connections:
  Pressure & Internal Energy Sensor (2P)/LConn1 -- A/RConn1
  Pressure & Internal Energy Sensor (2P)/RConn2 -- PS-S/LConn1
  Absolute Reference (2P)/LConn1 -- Pressure & Internal Energy Sensor (2P)/RConn1

== system ssc_Probes_2016a_org/TwoPhaseFluid/AbsTemp_2P ==
  PS-S : nesl_utility/PS-Simulink Converter  PhysicalDomain=network_engine_domain  SubClassName=ps_output  LeftPortType=input  RightPortType=output  PseudoPeriodic=off  Frequencies=[]  Unit=K  AffineConversion=off
  Terminator : Terminator
  Thermodynamic Properties Sensor (2P) : fl_lib/Two-Phase Fluid/Sensors/Thermodynamic Properties Sensor (2P)
      settings: SourceProductName=Simscape  SourceProductBaseCode=SS
  A : PMIOPort  Side=Left
  wires:
  [AbsTemp_2P] -> Terminator/1
  PS-S/1 -> [AbsTemp_2P]  "AbsTemp_2P"
  connections:
  Thermodynamic Properties Sensor (2P)/RConn1 -- PS-S/LConn1
  A/RConn1 -- Thermodynamic Properties Sensor (2P)/LConn1

== system ssc_Probes_2016a_org/TwoPhaseFluid/EnergyFlow_2P ==
  Mass & Energy Flow Sensor (2P) : fl_lib/Two-Phase Fluid/Sensors/Mass & Energy Flow Sensor (2P)
      settings: SourceProductName=Simscape  SourceProductBaseCode=SS
  PS-S : nesl_utility/PS-Simulink Converter  PhysicalDomain=network_engine_domain  SubClassName=ps_output  LeftPortType=input  RightPortType=output  PseudoPeriodic=off  Frequencies=[]  Unit=kW  AffineConversion=off
  Terminator : Terminator
  A : PMIOPort  Side=Left
  B : PMIOPort  Port=2  Side=Right
  wires:
  PS-S/1 -> [EnergyFlow_2P]  "EnergyFlow_2P"
  [EnergyFlow_2P] -> Terminator/1
  connections:
  Mass & Energy Flow Sensor (2P)/LConn1 -- A/RConn1
  Mass & Energy Flow Sensor (2P)/RConn3 -- PS-S/LConn1
  Mass & Energy Flow Sensor (2P)/RConn1 -- B/RConn1

== system ssc_Probes_2016a_org/TwoPhaseFluid/Enthalpy_2P ==
  PS-S : nesl_utility/PS-Simulink Converter  PhysicalDomain=network_engine_domain  SubClassName=ps_output  LeftPortType=input  RightPortType=output  PseudoPeriodic=off  Frequencies=[]  Unit=kJ/kg  AffineConversion=off
  Terminator : Terminator
  Thermodynamic Properties Sensor (2P) : fl_lib/Two-Phase Fluid/Sensors/Thermodynamic Properties Sensor (2P)
      settings: SourceProductName=Simscape  SourceProductBaseCode=SS
  A : PMIOPort  Side=Left
  wires:
  PS-S/1 -> [Enthalpy_2P]  "Enthalpy_2P"
  [Enthalpy_2P] -> Terminator/1
  connections:
  A/RConn1 -- Thermodynamic Properties Sensor (2P)/LConn1
  Thermodynamic Properties Sensor (2P)/RConn2 -- PS-S/LConn1

== system ssc_Probes_2016a_org/TwoPhaseFluid/InternalEnergy_2P ==
  Absolute Reference (2P) : fl_lib/Two-Phase Fluid/Elements/Absolute Reference (2P)
      settings: SourceProductName=Simscape  SourceProductBaseCode=SS
  PS-S : nesl_utility/PS-Simulink Converter  PhysicalDomain=network_engine_domain  SubClassName=ps_output  LeftPortType=input  RightPortType=output  PseudoPeriodic=off  Frequencies=[]  Unit=kJ/kg  AffineConversion=off
  Pressure & Internal Energy Sensor (2P) : fl_lib/Two-Phase Fluid/Sensors/Pressure & Internal Energy Sensor (2P)
      settings: SourceProductName=Simscape  SourceProductBaseCode=SS
  Terminator : Terminator
  A : PMIOPort  Side=Left
  wires:
  [InternalEnergy_2P] -> Terminator/1
  PS-S/1 -> [InternalEnergy_2P]  "InternalEnergy_2P"
  connections:
  Absolute Reference (2P)/LConn1 -- Pressure & Internal Energy Sensor (2P)/RConn1
  Pressure & Internal Energy Sensor (2P)/RConn3 -- PS-S/LConn1
  Pressure & Internal Energy Sensor (2P)/LConn1 -- A/RConn1

== system ssc_Probes_2016a_org/TwoPhaseFluid/MassFlow_2P ==
  Mass & Energy Flow Sensor (2P) : fl_lib/Two-Phase Fluid/Sensors/Mass & Energy Flow Sensor (2P)
      settings: SourceProductName=Simscape  SourceProductBaseCode=SS
  PS-S : nesl_utility/PS-Simulink Converter  PhysicalDomain=network_engine_domain  SubClassName=ps_output  LeftPortType=input  RightPortType=output  PseudoPeriodic=off  Frequencies=[]  Unit=kg/s  AffineConversion=off
  Terminator : Terminator
  A : PMIOPort  Side=Left
  B : PMIOPort  Port=2  Side=Right
  wires:
  [MassFlow_2P] -> Terminator/1
  PS-S/1 -> [MassFlow_2P]  "MassFlow_2P"
  connections:
  Mass & Energy Flow Sensor (2P)/RConn1 -- B/RConn1
  Mass & Energy Flow Sensor (2P)/RConn2 -- PS-S/LConn1
  Mass & Energy Flow Sensor (2P)/LConn1 -- A/RConn1

== system ssc_Probes_2016a_org/TwoPhaseFluid/SpecificVol_2P ==
  PS-S : nesl_utility/PS-Simulink Converter  PhysicalDomain=network_engine_domain  SubClassName=ps_output  LeftPortType=input  RightPortType=output  PseudoPeriodic=off  Frequencies=[]  Unit=m^3/kg  AffineConversion=off
  Terminator : Terminator
  Thermodynamic Properties Sensor (2P) : fl_lib/Two-Phase Fluid/Sensors/Thermodynamic Properties Sensor (2P)
      settings: SourceProductName=Simscape  SourceProductBaseCode=SS
  A : PMIOPort  Side=Left
  wires:
  [SpecificVol_2P] -> Terminator/1
  PS-S/1 -> [SpecificVol_2P]  "SpecificVol_2P"
  connections:
  Thermodynamic Properties Sensor (2P)/RConn3 -- PS-S/LConn1
  A/RConn1 -- Thermodynamic Properties Sensor (2P)/LConn1

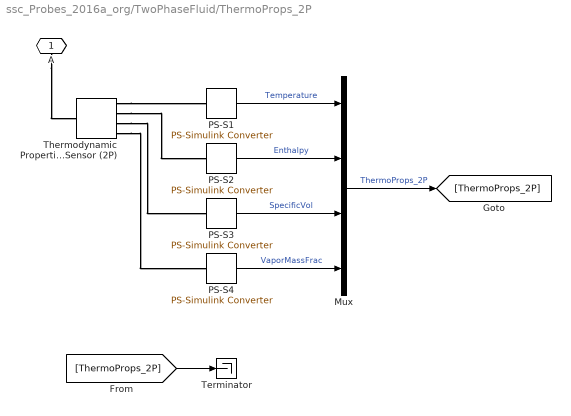
== system ssc_Probes_2016a_org/TwoPhaseFluid/ThermoProps_2P ==
  Mux : Mux
  PS-S1 : nesl_utility/PS-Simulink Converter  PhysicalDomain=network_engine_domain  SubClassName=ps_output  LeftPortType=input  RightPortType=output  PseudoPeriodic=off  Frequencies=[]  Unit=K  AffineConversion=off
  PS-S2 : nesl_utility/PS-Simulink Converter  PhysicalDomain=network_engine_domain  SubClassName=ps_output  LeftPortType=input  RightPortType=output  PseudoPeriodic=off  Frequencies=[]  Unit=kJ/kg  AffineConversion=off
  PS-S3 : nesl_utility/PS-Simulink Converter  PhysicalDomain=network_engine_domain  SubClassName=ps_output  LeftPortType=input  RightPortType=output  PseudoPeriodic=off  Frequencies=[]  Unit=m^3/kg  AffineConversion=off
  PS-S4 : nesl_utility/PS-Simulink Converter  PhysicalDomain=network_engine_domain  SubClassName=ps_output  LeftPortType=input  RightPortType=output  PseudoPeriodic=off  Frequencies=[]  Unit=1  AffineConversion=off
  Terminator : Terminator
  Thermodynamic Properties Sensor (2P) : fl_lib/Two-Phase Fluid/Sensors/Thermodynamic Properties Sensor (2P)
      settings: SourceProductName=Simscape  SourceProductBaseCode=SS
  A : PMIOPort  Side=Left
  wires:
  PS-S4/1 -> Mux/4  "VaporMassFrac"
  PS-S3/1 -> Mux/3  "SpecificVol"
  PS-S2/1 -> Mux/2  "Enthalpy"
  PS-S1/1 -> Mux/1  "Temperature"
  [ThermoProps_2P] -> Terminator/1
  Mux/1 -> [ThermoProps_2P]  "ThermoProps_2P"
  connections:
  Thermodynamic Properties Sensor (2P)/RConn4 -- PS-S4/LConn1
  Thermodynamic Properties Sensor (2P)/RConn3 -- PS-S3/LConn1
  Thermodynamic Properties Sensor (2P)/RConn2 -- PS-S2/LConn1
  Thermodynamic Properties Sensor (2P)/RConn1 -- PS-S1/LConn1
  A/RConn1 -- Thermodynamic Properties Sensor (2P)/LConn1

== system ssc_Probes_2016a_org/TwoPhaseFluid/VaporMassFraction_2P ==
  PS-S : nesl_utility/PS-Simulink Converter  PhysicalDomain=network_engine_domain  SubClassName=ps_output  LeftPortType=input  RightPortType=output  PseudoPeriodic=off  Frequencies=[]  Unit=1  AffineConversion=off
  Terminator : Terminator
  Thermodynamic Properties Sensor (2P) : fl_lib/Two-Phase Fluid/Sensors/Thermodynamic Properties Sensor (2P)
      settings: SourceProductName=Simscape  SourceProductBaseCode=SS
  A : PMIOPort  Side=Left
  wires:
  PS-S/1 -> [VaporMassFraction_2P]  "VaporMassFraction_2P"
  [VaporMassFraction_2P] -> Terminator/1
  connections:
  A/RConn1 -- Thermodynamic Properties Sensor (2P)/LConn1
  Thermodynamic Properties Sensor (2P)/RConn4 -- PS-S/LConn1

== system ssc_Probes_2016a_org/TwoPhaseFluid/VolumetricFlow_2P ==
  PS-S : nesl_utility/PS-Simulink Converter  PhysicalDomain=network_engine_domain  SubClassName=ps_output  LeftPortType=input  RightPortType=output  PseudoPeriodic=off  Frequencies=[]  Unit=m^3/s  AffineConversion=off
  Terminator : Terminator
  Volumetric Flow Sensor (2P) : fl_lib/Two-Phase Fluid/Sensors/Volumetric Flow Sensor (2P)
      settings: SourceProductName=Simscape  SourceProductBaseCode=SS
  A : PMIOPort  Side=Left
  B : PMIOPort  Port=2  Side=Right
  wires:
  [VolumetricFlow_2P] -> Terminator/1
  PS-S/1 -> [VolumetricFlow_2P]  "VolumetricFlow_2P"
  connections:
  Volumetric Flow Sensor (2P)/RConn1 -- B/RConn1
  Volumetric Flow Sensor (2P)/RConn2 -- PS-S/LConn1
  Volumetric Flow Sensor (2P)/LConn1 -- A/RConn1

== system ssc_Probes_2016a_org/TwoPhaseFluid/dEnergy_2P ==
  PS-S : nesl_utility/PS-Simulink Converter  PhysicalDomain=network_engine_domain  SubClassName=ps_output  LeftPortType=input  RightPortType=output  PseudoPeriodic=off  Frequencies=[]  Unit=kJ/kg  AffineConversion=off
  Pressure & Internal Energy Sensor (2P) : fl_lib/Two-Phase Fluid/Sensors/Pressure & Internal Energy Sensor (2P)
      settings: SourceProductName=Simscape  SourceProductBaseCode=SS
  Terminator : Terminator
  A : PMIOPort  Side=Left
  B : PMIOPort  Port=2  Side=Right
  wires:
  [dEnergy_2P] -> Terminator/1
  PS-S/1 -> [dEnergy_2P]  "dEnergy_2P"
  connections:
  Pressure & Internal Energy Sensor (2P)/LConn1 -- A/RConn1
  Pressure & Internal Energy Sensor (2P)/RConn1 -- B/RConn1
  Pressure & Internal Energy Sensor (2P)/RConn3 -- PS-S/LConn1

== system ssc_Probes_2016a_org/TwoPhaseFluid/dPressure_2P ==
  PS-S : nesl_utility/PS-Simulink Converter  PhysicalDomain=network_engine_domain  SubClassName=ps_output  LeftPortType=input  RightPortType=output  PseudoPeriodic=off  Frequencies=[]  Unit=Pa  AffineConversion=off
  Pressure & Internal Energy Sensor (2P) : fl_lib/Two-Phase Fluid/Sensors/Pressure & Internal Energy Sensor (2P)
      settings: SourceProductName=Simscape  SourceProductBaseCode=SS
  Terminator : Terminator
  A : PMIOPort  Side=Left
  B : PMIOPort  Port=2  Side=Right
  wires:
  PS-S/1 -> [dPressure_2P]  "dPressure_2P"
  [dPressure_2P] -> Terminator/1
  connections:
  Pressure & Internal Energy Sensor (2P)/RConn1 -- B/RConn1
  Pressure & Internal Energy Sensor (2P)/LConn1 -- A/RConn1
  Pressure & Internal Energy Sensor (2P)/RConn2 -- PS-S/LConn1
